simulink model "VnVShortestQueueAndProduct"  (R2018b)
settings: Solver=VariableStepAuto  StartTime=0.0  StopTime=11  RelTol=1e-3
undefined symbols (not defined in the file): m, n
settings Model: Creator=Ryan  LastModifiedBy=Ryan

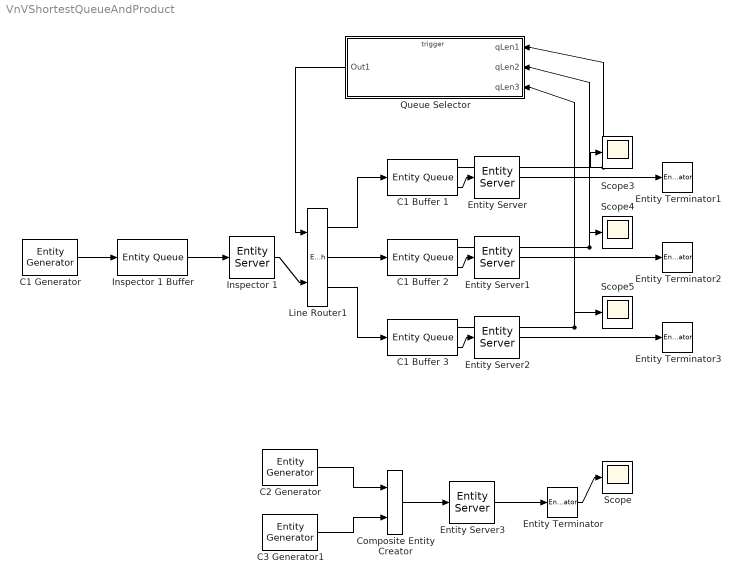
== system VnVShortestQueueAndProduct ==
  C1 Buffer 1 : EntityQueue  InputPortMessageModes=m  OutputPortMessageModes=n,m  NumberEntitiesInBlock=on
      settings: OutputPortMap=o1,o5
  C1 Buffer 2 : EntityQueue  InputPortMessageModes=m  OutputPortMessageModes=n,m  NumberEntitiesInBlock=on
      settings: OutputPortMap=o1,o5
  C1 Buffer 3 : EntityQueue  InputPortMessageModes=m  OutputPortMessageModes=n,m  NumberEntitiesInBlock=on
      settings: OutputPortMap=o1,o5
  C1 Generator : EntityGenerator  OutputPortMessageModes=m  Period=0  AttributeName=entityType|outputPort  AttributeInitialValue=1|1  EntityType=Structured  EntityTypeName=Entity
  C2 Generator : EntityGenerator  OutputPortMessageModes=m  Period=5  AttributeName=entityType|outputPort  AttributeInitialValue=2|1  EntityType=Structured  EntityTypeName=Entity
  C3 Generator1 : EntityGenerator  OutputPortMessageModes=m  Period=0  AttributeName=entityType|outputPort  AttributeInitialValue=3|1  EntityType=Structured  EntityTypeName=Entity
  Composite Entity Creator : CompositeEntityCreator  InputPortMessageModes=m,m  OutputPortMessageModes=m  EntityTypeName=Combined
      settings: InputPortMap=u0,u1
  Entity Server : EntityServer  InputPortMessageModes=m  OutputPortMessageModes=m  Capacity=1  ServiceTimeValue=20
  Entity Server1 : EntityServer  InputPortMessageModes=m  OutputPortMessageModes=m  Capacity=1  ServiceTimeValue=20
  Entity Server2 : EntityServer  InputPortMessageModes=m  OutputPortMessageModes=m  Capacity=1  ServiceTimeValue=20
  Entity Server3 : EntityServer  InputPortMessageModes=m  OutputPortMessageModes=m  Capacity=1
  Entity Terminator : EntityTerminator  InputPortMessageModes=m  NumberEntitiesArrived=on
      settings: OutputPortMap=o0
  Entity Terminator1 : EntityTerminator  InputPortMessageModes=m
  Entity Terminator2 : EntityTerminator  InputPortMessageModes=m
  Entity Terminator3 : EntityTerminator  InputPortMessageModes=m
  Inspector 1 : EntityServer  InputPortMessageModes=m  OutputPortMessageModes=m  Capacity=1  ServiceTimeAction=dt = wblrnd(10.725, 1.096);  EntryAction=|
      | % Entity will select the shortest queue
      | pickShortestQueue();
  Inspector 1 Buffer : EntityQueue  InputPortMessageModes=m  OutputPortMessageModes=m
      settings: OutputPortMap=o5
  Line Router1 : EntityOutputSwitch  InputPortMessageModes=m,m  OutputPortMessageModes=m,m,m  NumberOutputPorts=3  SwitchingCriterion=From control port  SwitchAttributeName=QueuePath
      settings: InputPortMap=u0,u1  OutputPortMap=o0,o1,o2
  Queue Selector : Subsystem  TreatAsAtomicUnit=on
  Scope{,3..5} (4 alike) : Scope
  wires:
  C1 Generator/1 -> Inspector 1 Buffer/1
  Inspector 1 Buffer/1 -> Inspector 1/1
  Inspector 1/1 -> Line Router1/2
  C1 Buffer 1/1 -> Queue Selector/1(qLen1), Scope3/1
  Line Router1/1 -> C1 Buffer 1/1
  Queue Selector/1(Out1) -> Line Router1/1
  C1 Buffer 3/1 -> Queue Selector/3(qLen3), Scope5/1
  Line Router1/2 -> C1 Buffer 2/1
  Line Router1/3 -> C1 Buffer 3/1
  C1 Buffer 2/1 -> Queue Selector/2(qLen2), Scope4/1
  C1 Buffer 1/2 -> Entity Server/1
  C1 Buffer 2/2 -> Entity Server1/1
  C1 Buffer 3/2 -> Entity Server2/1
  C2 Generator/1 -> Composite Entity Creator/1
  C3 Generator1/1 -> Composite Entity Creator/2
  Composite Entity Creator/1 -> Entity Server3/1
  Entity Server3/1 -> Entity Terminator/1
  Entity Terminator/1 -> Scope/1
  Entity Server/1 -> Entity Terminator1/1
  Entity Server1/1 -> Entity Terminator2/1
  Entity Server2/1 -> Entity Terminator3/1

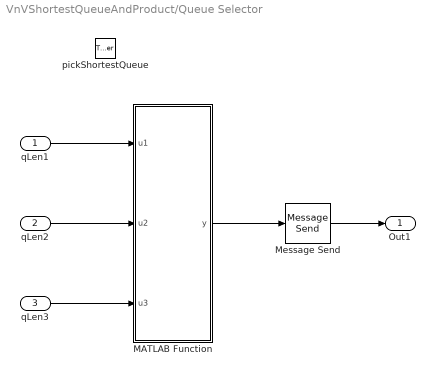
== system VnVShortestQueueAndProduct/Queue Selector ==
  qLen1 : Inport
  qLen2 : Inport  Port=2
  qLen3 : Inport  Port=3
  pickShortestQueue : TriggerPort  TriggerType=function-call  IsSimulinkFunction=on  FunctionName=pickShortestQueue  FunctionVisibility=scoped  VariantControl=Variant
  MATLAB Function : MATLAB Function  TreatAsAtomicUnit=on
  Message Send : MessageSend  OutputPortMessageModes=m
      settings: InputPortMap=u1
  Out1 : Outport
  wires:
  qLen1/1 -> MATLAB Function/1(u1)
  qLen2/1 -> MATLAB Function/2(u2)
  qLen3/1 -> MATLAB Function/3(u3)
  MATLAB Function/1(y) -> Message Send/1
  Message Send/1 -> Out1/1

== matlab function VnVShortestQueueAndProduct/Queue Selector/MATLAB Function ==
  data: u1 input; y output; u2 input; u3 input
function y = fcn(u1, u2, u3)
%#codegen

% Identify which input index is the smallest
[~,y] = min([u1 u2 u3]);
